simulink model "SimulationDemo"  (R2025b)
settings: Solver=ode4  StartTime=0.0  StopTime=200  FixedStep=0.02  RelTol=1e-3
InitFcn:
  | Initialization
model workspace (MAT data in the model file):
  actuatorInitial.Aileron_deg = 0
  actuatorInitial.Elevator_deg = 0
  actuatorInitial.Rudder_deg = 0
  contactParams.Kz_Npm = 5000
  contactParams.Cz_Nspm = 160
  contactParams.FrictionMu = 0.03
  contactParams.SlipSpeed_mps = 0.15
  contactParams.RampGain_1pm = 200
  contactParams.NormalScaleMax = 8
  contactParams.GroundPitch_rad = 0.0523598775598
  contactParams.PitchK_NmPerRad = -0.5
  contactParams.PitchC_NmPerRadps = -1
  contactParams.LateralFrictionMu = 1.5
  contactParams.RollK_NmPerRad = -8
  contactParams.RollC_NmPerRadps = -2.5
  contactParams.YawK_NmPerRad = -12
  contactParams.YawC_NmPerRadps = -4
  flightProtection.VMin_mps = 2
  flightProtection.VEps_mps = 0.001
  flightProtection.QGateBreakpoints_mps = [0 2 5]
  flightProtection.QGateTable = [0 0 1]
  flightProtection.BetaGateStartU_mps = 8
  flightProtection.BetaGateFullU_mps = 18
  initial.Heading = -2.35619449019
  initial.Roll = 0
  initial.Pitch = 0.0523598775598
  initial.Yaw = -2.35619449019
  initial.p = 0
  initial.q = 0.0001
  initial.r = 0.0001
  initial.u = 0.1
  initial.v = 0
  initial.w = 0.001
  initial.Altitude_MSL = 239
  initial.Altitude_AGL = 0
  initial.CGInertial.X = 0
  initial.CGInertial.Y = 0
  initial.CGInertial.Z = -239
  initial.Xe = [0 0 -239]
  initial.Mass.Empty = 1.67
  initial.Mass.Payload = 1.25
  initial.Mass.GrossTO = 2.92
  initial.Inertia = [0.026  0  0.0007; 0  0.072  0; 0.0007  0  0.096]
undefined symbols (not defined in the file): aeroData, aileronMax, aileronMin, dirPitch, dirRoll, dirThrottle, dirYaw, elevatorMax, elevatorMin, envActive, envCustomSource, envPresetSource, F, geometry, MIL, Moderate, pitchCh, pitchDB, propulsionData, rollCh, rollDB, throttleCh, throttleDB, uPitchMax, uPitchMin, uRollMax, uRollMin, uThrottleMax, uThrottleMin, uYawMax, uYawMin, yawCh, yawDB
libraries: simulink_extras x4, aerolibwind2 x3, aerolibasang x2, aerolibsim3d x2, aerolibadyn x1, matrix_library x1, sl3dlib x1, aerolibatmos2 x1, uavutilslib x1, sim3dlib x1
(part 1 of 2)
settings Model: DataDictionary=environmentData.sldd  Creator=klakhara  LastModifiedBy=klakhara
settings SolverCC: ODENIntegrationMethod=ode4

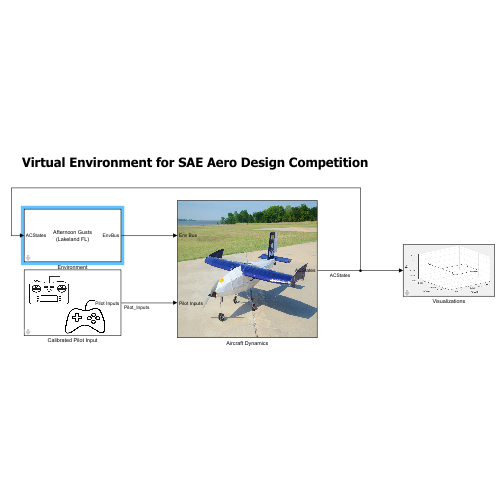
[thumbnail: Simulink's stored preview of the top-level diagram]
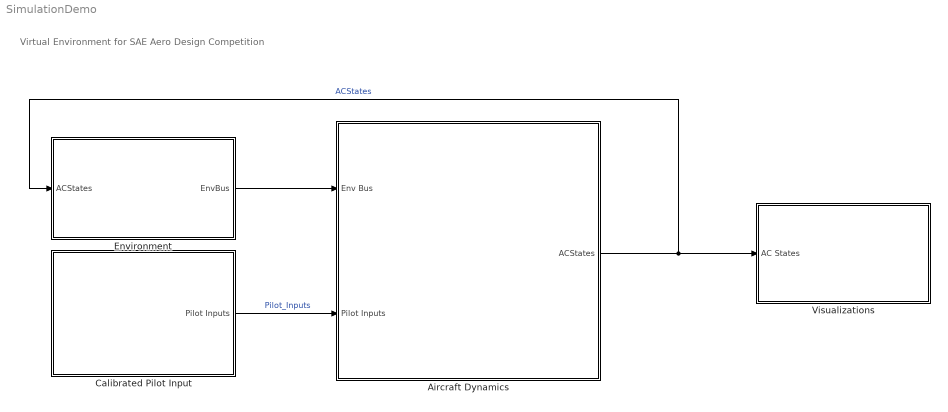
== system SimulationDemo ==
  note: Virtual Environment for SAE Aero Design Competition
  Aircraft Dynamics : Subsystem
      mask Display: image('Aircraft.jpg');
  Calibrated Pilot Input : Subsystem  mask{configName=0, joystickID=Joystick1}
      mask prompts: joystickID "Device ID:"
      mask TypeOptions joystickID: None | Joystick1 | Joystick2 | Joystick3 | Joystick4 | Joystick5 | Joystick6 | Joystick7 | Joystick8 | Joystick9 | Joystick10 | Joystick11 | Joystick12
      mask DialogControl DescGroupVar Prompt: Import calibration parameters to setup the calibreated input device
      mask DialogControl DescTextVar Prompt: Import your calibration configuration file:
      mask DialogControl loadConfig Prompt: Load file
      mask DialogControl ParameterGroupVar Prompt: Identify your Pilot Input Device:
      mask Display: image('Controller_Setup.jpg');
  Environment : Subsystem  mask(SAE Aero Environment){envPreset=Afternoon Gusts - Lakeland FL (2.0x), customName=VIT Vellore, customDescription=VIT Vellore, customMultiplier=1, customCompetitionSite=off, customLocationName=Custom Site, customCity=, customCountry=, customLatitude_deg=0, customLongitude_deg=0, customElevation_MSL_m=0, customAtmosphereElevation_MSL_m=0, customISADeviation_C=0, customTemperature_C=15, customPressure_Pa=101325, customDensity_kgm3=1.225, customWindShearSpeed_mps=0, customWindShearDirection_deg=0, customWindShearExponent=0.143, customTurbulenceOn=off, customTurbulenceSpeed_mps=0, customTurbulenceDirection_deg=0, customTurbulenceSigma_mps=0, customTurbulenceScale_m=205, customNoiseSeeds=[23341 23342 23343 23344], customGustEnableU=off, customGustEnableV=off, customGustEnableW=off, customGustAmplitude_mps=[0 0 0], customGustLength_m=[1 1 1], customGustStartTime_s=Inf, customGustStartAltitude_AGL_m=0}
      mask prompts: envPreset "Environment"; customName "Name"; customDescription "Description"; customMultiplier "Score multiplier"; customCompetitionSite "Competition site"; customLocationName "Location name"; customCity "City"; customCountry "Country or region"; customLatitude_deg "Latitude [deg]"; customLongitude_deg "Longitude [deg]"; customElevation_MSL_m "Elevation MSL [m]"; customAtmosphereElevation_MSL_m "Reference elevation [m]"; customISADeviation_C "ISA deviation [deg C]"; customTemperature_C "Temperature [deg C]"; customPressure_Pa "Pressure [Pa]"; customDensity_kgm3 "Density [kg/m^3]"; customWindShearSpeed_mps "Speed at 6 m [m/s]"; customWindShearDirection_deg "Direction [deg]"; customWindShearExponent "Power-law exponent"; customTurbulenceOn "Enable turbulence"; customTurbulenceSpeed_mps "Speed at 6 m [m/s]"; customTurbulenceDirection_deg "Direction [deg]"; customTurbulenceSigma_mps "Sigma [m/s]"; customTurbulenceScale_m "Scale length [m]"; customNoiseSeeds "Noise seeds [1x4]"; customGustEnableU "Enable U-axis gust"; customGustEnableV "Enable V-axis gust"; customGustEnableW "Enable W-axis gust"; customGustAmplitude_mps "Amplitude [u v w] m/s"; customGustLength_m "Length [dx dy dz] m"; customGustStartTime_s "Start time [s]"; customGustStartAltitude_AGL_m "Start altitude AGL [m]"
      mask help: Select a predefined environment or enter a complete custom environment definition.
      mask init:
      | EnvironmentMask.initialize(gcb);
      mask TypeOptions envPreset: Custom environment | Sea Level Standard (1.0x) | Aero Design West - Van Nuys CA (1.1x) | Aero Design East FL - Lakeland (1.2x) | Aero Design East TX - Fort Worth (1.3x) | Hot Day - Chennai India (1.5x) | Cold Windy Day - Toronto (1.6x) | Afternoon Gusts - Lakeland FL (2.0x) | High Altitude - Denver-type (2.5x)
      mask Callback envPreset: EnvironmentMask.selectionChanged(gcb);
      mask DialogControl Container1 Prompt: Environment source
      mask DialogControl Control1 Prompt: Predefined environments are loaded from environmentData.sldd.
      mask DialogControl envPreset Tooltip: Choose a catalog environment or enter a custom definition.
      mask DialogControl customGeneralTab Prompt: General
      mask DialogControl customName Tooltip: Name stored with simulation environment metadata.
      mask DialogControl customDescription Tooltip: Description stored with the environment.
      mask DialogControl customMultiplier Tooltip: Positive mission score multiplier.
      mask DialogControl customCompetitionSite Tooltip: Marks this environment as an official competition site.
      mask DialogControl customLocationTab Prompt: Location
      mask DialogControl customLocationName Tooltip: Airfield or test-site name.
      mask DialogControl customCity Tooltip: Location city.
      mask DialogControl customCountry Tooltip: Location country or region.
      mask DialogControl customLatitude_deg Tooltip: Geodetic latitude from -90 to 90 degrees.
      mask DialogControl customLongitude_deg Tooltip: Longitude from -180 to 180 degrees.
      mask DialogControl customElevation_MSL_m Tooltip: Site elevation above mean sea level.
      mask DialogControl customAtmosphereTab Prompt: Atmosphere
      mask DialogControl customAtmosphereElevation_MSL_m Tooltip: Elevation associated with the atmospheric measurements.
      mask DialogControl customISADeviation_C Tooltip: Temperature difference from ISA.
      mask DialogControl customTemperature_C Tooltip: Measured or specified air temperature.
      mask DialogControl customPressure_Pa Tooltip: Positive static air pressure.
      mask DialogControl customDensity_kgm3 Tooltip: Positive air density.
      mask DialogControl customWindTab Prompt: Wind shear
      mask DialogControl customWindShearSpeed_mps Tooltip: Nonnegative wind speed at the reference height.
      mask DialogControl customWindShearDirection_deg Tooltip: Meteorological direction clockwise from north.
      mask DialogControl customWindShearExponent Tooltip: Positive terrain-dependent shear exponent.
      mask DialogControl customTurbulenceTab Prompt: Turbulence
      mask DialogControl customTurbulenceOn Tooltip: Enable the Dryden turbulence model.
      mask DialogControl customTurbulenceSpeed_mps Tooltip: Nonnegative mean wind speed used by Dryden turbulence.
      mask DialogControl customTurbulenceDirection_deg Tooltip: Direction clockwise from north.
      mask DialogControl customTurbulenceSigma_mps Tooltip: RMS turbulence intensity.
      mask DialogControl customTurbulenceScale_m Tooltip: Positive medium/high-altitude scale length.
      mask DialogControl customNoiseSeeds Tooltip: Four nonnegative integer seeds.
      mask DialogControl customGustTab Prompt: Gust
      mask DialogControl customGustEnableU Tooltip: Enable longitudinal gust.
      mask DialogControl customGustEnableV Tooltip: Enable lateral gust.
      mask DialogControl customGustEnableW Tooltip: Enable vertical gust.
      mask DialogControl customGustAmplitude_mps Tooltip: Three gust velocity components.
      mask DialogControl customGustLength_m Tooltip: Three positive gust wavelengths.
      mask DialogControl customGustStartTime_s Tooltip: Nonnegative gust start time; use Inf to disable by time.
      mask DialogControl customGustStartAltitude_AGL_m Tooltip: Nonnegative gust onset altitude.
      mask Display:
      | try
      |     disp(EnvironmentMask.formatIconLabel(environmentName));
      | catch
      |     disp('Environment');
      | end
  Visualizations : Subsystem  mask{visualization=3D Animation, FlightParam=on}
      mask prompts: visualization "Trajectory visualization"; FlightParam "Plot flight parameters"
      mask Callback FlightParam:
      | scopeBlocks = find_system(gcb, 'LookUnderMasks', 'all', 'FollowLinks', 'off', 'MatchFilter', @Simulink.match.allVariants, 'BlockType', 'Scope');
      | scopeState = get_param(gcb, 'FlightParam');
      | for scopeIndex = 1:numel(scopeBlocks)
      |     set_param(scopeBlocks{scopeIndex}, 'OpenAtSimulationStart', scopeState, 'Open', scopeState);
      | end
      | clear scopeBlocks scopeState scopeIndex
      mask DialogControl DescTextVar Prompt: Select your visualization type and if you want to plot flight paramets in scope.
      mask Display:
      | % Get selected variant from mask
      | v = get_param(gcb, 'visualization');
      | 
      | 
      | % Choose image based on variant
      | switch v
      |     case '3D Animation'
      |         img = imread('3D_Animation.png');
      |         image(img);
      |         % axis off
      |         % axis image
      |     case "Unreal Engine"
      |         img = imread('Unreal_Engine.png');
      |         image(img);
      |         % axis off
      |         % axis image
      |     case 'Off'
      |         % No image
      | 
      | end
      | 
      | % Display image as block icon
  wires:
  Aircraft Dynamics/1(ACStates) -> Visualizations/1(AC States), Environment/1(ACStates)  "ACStates"
  Environment/1(EnvBus) -> Aircraft Dynamics/1(Env Bus)
  Calibrated Pilot Input/1(Pilot Inputs) -> Aircraft Dynamics/2(Pilot Inputs)  "Pilot_Inputs"

== system SimulationDemo/Aircraft Dynamics ==
  Env Bus : Inport
  Pilot Inputs : Inport  Port=2
  ACStates To Workspace : ToWorkspace  VariableName=ACStates  SaveFormat=Timeseries  SampleTime=-1
  Actuator Dynamics : Subsystem
  Bus Creator : BusCreator  Inputs=8
  Bus Selector : BusSelector  OutputSignals=Actuator deflections
  Equation of motion : EOM6DOFBodyQuat  xme_0=initial.Xe  Vm_0=[initial.u initial.v initial.w]  eul_0=[initial.Roll initial.Pitch initial.Yaw]  pm_0=[initial.p initial.q initial.r]  mass_0=initial.Mass.GrossTO  inertia=initial.Inertia
  Flight Parameters : Subsystem
  Forces & Moments : Subsystem
  Gain : Gain  Gain=[1, 1, -1]
  ACStates : Outport
  wires:
  Actuator Dynamics/1(Actuator_Deflections) -> Bus Creator/8, Forces & Moments/4(Pilot_Inputs)  "Actuator deflections"
  Bus Selector/1 -> Actuator Dynamics/1(Actuator_Command)  "<Actuator deflections>"
  Pilot Inputs/1 -> Bus Selector/1  "Pilot_Inputs"
  Forces & Moments/2(Moments) -> Equation of motion/2
  Forces & Moments/1(Forces) -> Equation of motion/1
  Flight Parameters/1(Flight_Parameters) -> Forces & Moments/2(Flight Params)
  Equation of motion/2 -> Gain/1
  Equation of motion/4 -> Bus Creator/4  "q"
  Gain/1 -> Bus Creator/2  "Xe"
  Env Bus/1 -> Flight Parameters/2(EnvirBus), Forces & Moments/3(Env Bus)
  Equation of motion/1 -> Bus Creator/1  "Ve"
  Equation of motion/5 -> Bus Creator/5  "DCM_be"
  Equation of motion/7 -> Bus Creator/7  "wb"
  Equation of motion/6 -> Bus Creator/6  "Vb"
  Equation of motion/3 -> Bus Creator/3  "Euler_angles"
  Bus Creator/1 -> Forces & Moments/1(States), Flight Parameters/1("AC States "), ACStates To Workspace/1, ACStates/1  "ACStates"

== system SimulationDemo/Calibrated Pilot Input ==
  Actuator scaling : Subsystem
  Bus Creator : BusCreator  Inputs=2
  PilotInput : BusCreator  Inputs=4
  Simulation 3D Joystick : sl3dlib/Simulation 3D/Hardware Interface/Simulation 3D Joystick  joyid=1  adjustports=on  forcefeed=off
  Terminator : Terminator
  Pilot Inputs : Outport
  wires:
  Bus Creator/1 -> Pilot Inputs/1
  Simulation 3D Joystick/1 -> Bus Creator/1, Actuator scaling/1(In1)  "Raw Inputs"
  Actuator scaling/2(Elevator) -> PilotInput/2  "Elevator"
  Simulation 3D Joystick/2 -> Terminator/1
  PilotInput/1 -> Bus Creator/2  "Actuator deflections"
  Actuator scaling/3(Rudder) -> PilotInput/3  "Rudder"
  Actuator scaling/4(Throttle) -> PilotInput/4  "Throttle"
  Actuator scaling/1(Aileron) -> PilotInput/1  "Aileron"

== system SimulationDemo/Environment ==
  ACStates : Inport
  AltitudeAGL : Sum  Inputs=+-
  AltitudeMSLValid : Saturate  UpperLimit=84852  LowerLimit=0
  AltitudePos : Gain  Gain=-1
  Bus Creator : BusCreator  Inputs=4
  Bus Creator1 : BusCreator  Inputs=2
  Bus Selector1 : BusSelector  OutputSignals=Xe,Ve,DCM_be
  Dot Product : DotProduct  OutDataTypeStr=Inherit: Inherit via internal rule
  Environment Source : Subsystem  Variant=on
  Mux : Mux  Inputs=3
  Reshape : Reshape  OutputDimensionality=Row vector (2-D)
  Selector2 : Selector  IndexMode=Zero-based  InputPortWidth=3  IndexOptions=Index vector (dialog)  Indices=2  OutputSizes=1
  Sqrt : Sqrt
  Temperature Adjusted Density : Subsystem
  "WGS84 Gravity Model  " : GravityWGS84  action=None
  Wind Models : Subsystem
  EnvBus : Outport  VectorParamsAs1DForOutWhenUnconnected=off
  wires:
  Wind Models/2(pg,qg,rg) -> Bus Creator1/2  "pqr_wind"
  Wind Models/1(ug,vg,wg) -> Bus Creator1/1  "uvw_wind"
  Bus Creator1/1 -> Bus Creator/4  "Vwind"
  Dot Product/1 -> Sqrt/1
  Sqrt/1 -> Wind Models/2(Airspeed)
  Bus Creator/1 -> EnvBus/1
  ACStates/1 -> Bus Selector1/1
  Bus Selector1/2 -> Dot Product/1, Dot Product/2  "<Ve>"
  Mux/1 -> Bus Creator/2, Reshape/1  "X"
  "WGS84 Gravity Model  "/1 -> Bus Creator/1  "g"
  Reshape/1 -> "WGS84 Gravity Model  "/1
  Bus Selector1/3 -> Wind Models/3(DCM)  "<DCM_be>"
  Bus Selector1/1 -> Selector2/1  "<Xe>"
  Selector2/1 -> AltitudePos/1
  AltitudeAGL/1 -> Wind Models/1(Altitude)
  AltitudePos/1 -> AltitudeMSLValid/1
  AltitudeMSLValid/1 -> Mux/3, AltitudeAGL/1, Temperature Adjusted Density/2(Height)
  Temperature Adjusted Density/1(rho) -> Bus Creator/3
  Environment Source/1(Latitude_deg) -> Mux/1  "Latitude_deg"
  Environment Source/2(Longitude_deg) -> Mux/2  "Longitude_deg"
  Environment Source/4(Elevation_MSL_m) -> AltitudeAGL/2  "Elevation_MSL_m"
  Environment Source/3(ISA_Deviation_C) -> Temperature Adjusted Density/1(ISA_Deviation_C)  "ISA_Deviation_C"

== system SimulationDemo/Visualizations ==
  AC States : Inport
  "Flight parameters " : Subsystem  Variant=on  EmptyChoice=on
  Trajectory Visualization : Subsystem  Variant=on  EmptyChoice=on
  wires:
  AC States/1 -> Trajectory Visualization/1(AC States), "Flight parameters "/1(In1)

== system SimulationDemo/Aircraft Dynamics/Actuator Dynamics ==
  Actuator_Command : Inport
  Aileron_Command_Limit : Saturate  UpperLimit=geometry.AileronLimit(2)  LowerLimit=geometry.AileronLimit(1)
  Aileron_Deflection_Limit : Saturate  UpperLimit=geometry.AileronLimit(2)  LowerLimit=geometry.AileronLimit(1)
  Aileron_Lag_0p05s : StateSpace  A=-20  B=20  D=0  InitialCondition=actuatorInitial.Aileron_deg
  Aileron_Rate_300dps : RateLimiter  RisingSlewLimit=300  FallingSlewLimit=-300  InitialCondition=actuatorInitial.Aileron_deg
  Command_Select : BusSelector  OutputSignals=Aileron,Elevator,Rudder,Throttle
  Deflection_Bus : BusCreator  Inputs=4
  Elevator_Command_Limit : Saturate  UpperLimit=geometry.ElevatorLimit(2)  LowerLimit=geometry.ElevatorLimit(1)
  Elevator_Deflection_Limit : Saturate  UpperLimit=geometry.ElevatorLimit(2)  LowerLimit=geometry.ElevatorLimit(1)
  Elevator_Lag_0p05s : StateSpace  A=-20  B=20  D=0  InitialCondition=actuatorInitial.Elevator_deg
  Elevator_Rate_300dps : RateLimiter  RisingSlewLimit=300  FallingSlewLimit=-300  InitialCondition=actuatorInitial.Elevator_deg
  Rudder_Command_Limit : Saturate  UpperLimit=geometry.RudderLimit(2)  LowerLimit=geometry.RudderLimit(1)
  Rudder_Deflection_Limit : Saturate  UpperLimit=geometry.RudderLimit(2)  LowerLimit=geometry.RudderLimit(1)
  Rudder_Lag_0p05s : StateSpace  A=-20  B=20  D=0  InitialCondition=actuatorInitial.Rudder_deg
  Rudder_Rate_300dps : RateLimiter  RisingSlewLimit=300  FallingSlewLimit=-300  InitialCondition=actuatorInitial.Rudder_deg
  Actuator_Deflections : Outport
  wires:
  Actuator_Command/1 -> Command_Select/1
  Aileron_Command_Limit/1 -> Aileron_Lag_0p05s/1
  Command_Select/1 -> Aileron_Command_Limit/1  "<Aileron>"
  Command_Select/2 -> Elevator_Command_Limit/1  "<Elevator>"
  Command_Select/3 -> Rudder_Command_Limit/1  "<Rudder>"
  Elevator_Command_Limit/1 -> Elevator_Lag_0p05s/1
  Command_Select/4 -> Deflection_Bus/4  "<Throttle>"
  Rudder_Command_Limit/1 -> Rudder_Lag_0p05s/1
  Aileron_Lag_0p05s/1 -> Aileron_Rate_300dps/1
  Elevator_Lag_0p05s/1 -> Elevator_Rate_300dps/1
  Rudder_Lag_0p05s/1 -> Rudder_Rate_300dps/1
  Aileron_Rate_300dps/1 -> Aileron_Deflection_Limit/1
  Elevator_Rate_300dps/1 -> Elevator_Deflection_Limit/1
  Rudder_Rate_300dps/1 -> Rudder_Deflection_Limit/1
  Elevator_Deflection_Limit/1 -> Deflection_Bus/2  "Elevator"
  Aileron_Deflection_Limit/1 -> Deflection_Bus/1  "Aileron"
  Rudder_Deflection_Limit/1 -> Deflection_Bus/3  "Rudder"
  Deflection_Bus/1 -> Actuator_Deflections/1

== system SimulationDemo/Aircraft Dynamics/Flight Parameters ==
  "AC States " : Inport
  EnvirBus : Inport  Port=2
  Bus Creator : BusCreator  Inputs=6
  Bus Selector1 : BusSelector  OutputSignals=rho
  Bus Selector2 : BusSelector  OutputSignals=Vb
  Bus Selector3 : BusSelector  OutputSignals=wb
  Bus Selector4 : BusSelector  OutputSignals=Vwind.uvw_wind,Vwind.pqr_wind
  Flight Parameters To Workspace : ToWorkspace  VariableName=FlightParameters  SaveFormat=Timeseries  SampleTime=-1
  "Incidence, Sideslip, & Airspeed" : aerolibasang/Incidence, Sideslip, & Airspeed
  Radians to Degrees : simulink_extras/Transformations/Radians to Degrees
  Radians to Degrees1 : simulink_extras/Transformations/Radians to Degrees
  Subsystem : Subsystem
      settings: PortSchema="{\"entries\":[{\"content\":{\"sides\":[{\"content\":{\"connectorIds\":[\"In1\",\"In2\"]},\"type\":\"ConnectorPlacement.EquallySpacedRectSide\",\"uuid\":\"5a143d0f-2436-4fb0-bb97-2c4984d07975\"},{\"content\":{\"connectorIds\":[\"Out1\"],\"side\":\"RIGHT\"},\"type\":\"ConnectorPlacement.EquallySpacedRectSide\",\"uuid\":\"8d58a2ee-82c7-4615-9bab-8cc4c0d46ad5\"},{\"content\":{\"connectorIds\":[\"In3\"],\"side\":\"TOP\"},\"type\":\"ConnectorPlacement.EquallySpacedRectSide\",\"uuid\":\"18f756c1-07a2-4df5-83f0-d5c22876817a\"}]},\"type\":\"ConnectorPlacement.EquallySpacedConnector\",\"uuid\":\"42d60932-45cf-443a-a7ca-3ff9305e2569\"}],\"packageUris\":[\"http://schema.mathworks.com/mf0/Connector/R2020b\"],\"version\":\"1.0\"}"
  Sum2 : Sum  InputSameDT=on  SaturateOnIntegerOverflow=on  OutDataTypeStr=Inherit: Same as first input
  Sum4 : Sum  Inputs=+-|  InputSameDT=on  SaturateOnIntegerOverflow=on  OutDataTypeStr=Inherit: Same as first input
  Vrel_safe : Subsystem
  Flight_Parameters : Outport  VectorParamsAs1DForOutWhenUnconnected=off
  wires:
  "AC States "/1 -> Bus Selector2/1, Bus Selector3/1
  Sum2/1 -> Bus Creator/5  "pqr_tot"
  Sum4/1 -> Vrel_safe/1(Vrel)  "Vrel"
  Bus Selector3/1 -> Sum2/2  "<wb>"
  EnvirBus/1 -> Bus Selector1/1, Bus Selector4/1
  Bus Selector2/1 -> Sum4/1  "<Vb>"
  Bus Selector4/2 -> Sum2/1  "<pqr_wind>"
  Bus Selector4/1 -> Sum4/2  "<uvw_wind>"
  "Incidence, Sideslip, & Airspeed"/3 -> Subsystem/3(TAS), Bus Creator/4  "TAS"
  "Incidence, Sideslip, & Airspeed"/1 -> Radians to Degrees/1
  "Incidence, Sideslip, & Airspeed"/2 -> Radians to Degrees1/1
  Vrel_safe/1(Vrel_safe) -> Subsystem/1(Vrel_safe), "Incidence, Sideslip, & Airspeed"/1, Bus Creator/1  "Vrel"
  Bus Selector1/1 -> Subsystem/2(<rho>)  "<rho>"
  Subsystem/1(q) -> Bus Creator/6  "dynamic Pressure"
  Radians to Degrees/1 -> Bus Creator/2  "alpha"
  Radians to Degrees1/1 -> Bus Creator/3  "beta"
  Bus Creator/1 -> Flight Parameters To Workspace/1, Flight_Parameters/1

== system SimulationDemo/Aircraft Dynamics/Forces & Moments ==
  note: Forces & Moments
      | 1. Gravitational Forces
      | 2. Aerodynamic Forces & Moments
      | 3. Propulsion Forces & Moments
  States : Inport
  Flight Params : Inport  Port=2
  Env Bus : Inport  Port=3
  Pilot_Inputs : Inport  Port=4
  Aerodynamic Forces & Moments : Subsystem
  Bus Selector : BusSelector  OutputSignals=g
  Bus Selector1 : BusSelector  OutputSignals=Xe,DCM_be,Vb
  Contact Forces & Moments : Subsystem
  Gravitational Forces : Subsystem
  Propulsion Forces & Moments : Subsystem
  Sum : Sum  Inputs=++++
  Sum1 : Sum  Inputs=+++
  Forces : Outport
  Moments : Outport  Port=2
  wires:
  Bus Selector1/3 -> Contact Forces & Moments/4(Vb)  "<Vb>"
  Contact Forces & Moments/1(F_Contact) -> Sum/4
  Bus Selector1/1 -> Contact Forces & Moments/2(Xe)  "<Xe>"
  Bus Selector1/2 -> Gravitational Forces/1(DCM)  "<DCM_be>"
  Sum1/1 -> Moments/1  "Moments"
  Sum/1 -> Forces/1  "Forces"
  Propulsion Forces & Moments/1(Forces_Propulsion) -> Sum/3  "F_Prop"
  Aerodynamic Forces & Moments/1(Forces_aero) -> Sum/2  "F_Aero"
  Gravitational Forces/1(Fgrav) -> Sum/1, Contact Forces & Moments/3(F_Gravity)  "F_Gravity"
  Bus Selector/1 -> Gravitational Forces/2(g)  "<g>"
  States/1 -> Bus Selector1/1, Contact Forces & Moments/1(States)  "States"
  Env Bus/1 -> Propulsion Forces & Moments/2(EnvBus), Bus Selector/1
  Flight Params/1 -> Aerodynamic Forces & Moments/1(Flight Params)
  Propulsion Forces & Moments/2(Moments_Propulsion) -> Sum1/2  "M_Prop"
  Pilot_Inputs/1 -> Aerodynamic Forces & Moments/2(Pilot_Input), Propulsion Forces & Moments/1(Pilot Inputs)
  Aerodynamic Forces & Moments/2(Moments_aero) -> Sum1/1  "M_Aero"
  Contact Forces & Moments/2(M_Contact) -> Sum1/3  "M_Contact"

== system SimulationDemo/Calibrated Pilot Input/Actuator scaling ==
  In1 : Inport
  Aileron Scaling : Subsystem
  Demux : Demux
  Elevator Scaling : Subsystem
  Rudder Scaling : Subsystem
  Selector : Selector  InputPortWidth=8  IndexOptions=Index vector (dialog)  Indices=[rollCh pitchCh yawCh throttleCh]  OutputSizes=1
  Throttle Scaling : Subsystem
  Aileron : Outport
  Elevator : Outport  Port=2
  Rudder : Outport  Port=3
  Throttle : Outport  Port=4
  wires:
  In1/1 -> Selector/1
  Rudder Scaling/1(actuator deflection) -> Rudder/1
  Demux/3 -> Rudder Scaling/1(raw signal)  "Yaw"
  Demux/1 -> Aileron Scaling/1(raw signal)  "roll"
  Selector/1 -> Demux/1
  Elevator Scaling/1(actuator deflection) -> Elevator/1
  Demux/4 -> Throttle Scaling/1(raw signal)  "Throttle"
  Demux/2 -> Elevator Scaling/1(raw signal)  "Pitch"
  Aileron Scaling/1(actuator deflection) -> Aileron/1
  Throttle Scaling/1(actuator deflection) -> Throttle/1

== system SimulationDemo/Environment/Environment Source ==
  note: 1) Add Subsystem or Model blocks as valid variant choices.
      | 2) You cannot connect blocks at this level. At simulation, connectivity is automatically
      | determined, based on the active variant and port name matching.
  Custom Environment Parameters : Subsystem  VariantControl=environmentSourceMode == 1
  Preset Environment Parameters : Subsystem  VariantControl=environmentSourceMode == 2
  Latitude_deg : Outport
  Longitude_deg : Outport  Port=2
  ISA_Deviation_C : Outport  Port=3
  Elevation_MSL_m : Outport  Port=4

== system SimulationDemo/Environment/Temperature Adjusted Density ==
  ISA_Deviation_C : Inport
  Height : Inport  Port=2
  Adjusted Temperature : Sum
  COESA Atmosphere Model : aerolibatmos2/COESA Atmosphere Model  units=Metric (MKS)  spec=1976 COESA-extended U.S. Standard Atmosphere  model=Profile  profile_var=High temperature  profile_percent=1%  profile_alt=5 km (16404 ft)  envelope_var=High temperature  envelope_percent=1%  action=Warning
  Density Correction : Product  Inputs=**/
  Temperature Guard : Saturate  UpperLimit=inf  LowerLimit=1
  Terminator2 : Terminator
  Terminator3 : Terminator
  rho : Outport
  wires:
  Adjusted Temperature/1 -> Temperature Guard/1
  COESA Atmosphere Model/3 -> Terminator2/1  "ps"
  COESA Atmosphere Model/1 -> Density Correction/2, Adjusted Temperature/2  "T"
  COESA Atmosphere Model/4 -> Density Correction/1  "rho"
  COESA Atmosphere Model/2 -> Terminator3/1  "a"
  Temperature Guard/1 -> Density Correction/3
  Height/1 -> COESA Atmosphere Model/1
  Density Correction/1 -> rho/1  "rho"
  ISA_Deviation_C/1 -> Adjusted Temperature/1

== system SimulationDemo/Environment/Wind Models ==
  Altitude : Inport  Unit=meter
  Airspeed : Inport  Port=2  Unit=m/s
  DCM : Inport  Port=3
  "DCM " : InportShadow  Port=3
  Discrete Wind Gust Model : aerolibwind2/Discrete Wind Gust Model  units=Metric (MKS)  Gx=off  Gy=on  Gz=off  t_0=envActive.Gust.StartTime_s  d_m=envActive.Gust.Length_m  v_m=envActive.Gust.Amplitude_mps
  Dryden Wind Turbulence Model (Continuous (+q -r)) : aerolibwind2/Dryden Wind Turbulence Model  (Continuous (+q -r))  units=Metric (MKS)  spec=MIL-F-8785C  model=Continuous Dryden (+q -r)  W20=envActive.Turbulence.Speed_6m_mps  Wdeg=envActive.Turbulence.Direction_deg  TurbProb=10^-3 - Moderate  L_high=envActive.Turbulence.Scale_Lu_m  Wingspan=geometry.Span  ts=0.5  Seed=envActive.Turbulence.NoiseSeeds  T_on=on
  Sum : Sum  Inputs=+++  InputSameDT=on  SaturateOnIntegerOverflow=on  OutDataTypeStr=Inherit: Same as first input
  Wind Shear Model : aerolibwind2/Wind Shear Model  units=Metric (MKS)  phase=Category C - Terminal Flight Phase  W_20=envActive.WindShear.Speed_6m_mps  Wdeg=envActive.WindShear.Direction_deg
  ug,vg,wg : Outport  Unit=m/s  VectorParamsAs1DForOutWhenUnconnected=off
  pg,qg,rg : Outport  Port=2  Unit=rad/second  VectorParamsAs1DForOutWhenUnconnected=off
  wires:
  "DCM "/1 -> Dryden Wind Turbulence Model (Continuous (+q -r))/3
  Wind Shear Model/1 -> Sum/1
  Dryden Wind Turbulence Model (Continuous (+q -r))/1 -> Sum/2
  Discrete Wind Gust Model/1 -> Sum/3
  Sum/1 -> ug,vg,wg/1
  DCM/1 -> Wind Shear Model/2
  Airspeed/1 -> Dryden Wind Turbulence Model (Continuous (+q -r))/2, Discrete Wind Gust Model/1
  Dryden Wind Turbulence Model (Continuous (+q -r))/2 -> pg,qg,rg/1
  Altitude/1 -> Dryden Wind Turbulence Model (Continuous (+q -r))/1, Wind Shear Model/1

== system SimulationDemo/Visualizations/Flight parameters  ==
  In1 : Inport
  Scope Plot : Subsystem  TreatAsAtomicUnit=on  VariantControl=FlightParam ==1

== system SimulationDemo/Visualizations/Trajectory Visualization ==
  AC States : Inport
  3D Animation : Subsystem  VariantControl="visualization == \"3D Animation\""
      mask Display: image('3D_Animation.png');
  Unreal Engine : Subsystem  VariantControl="visualization == \"Unreal Engine\""
      mask Display: image('Unreal_Engine.png');

== system SimulationDemo/Aircraft Dynamics/Flight Parameters/Subsystem ==
  note: Note: 1D lookup table here is used as a switch to protect dynamic pressure for speed below 2 m/sec and gradually ramps up till 5 m/sec.
  Vrel_safe : Inport
  <rho> : Inport  Port=2
  TAS : Inport  Port=3
  1-D Lookup Table : Lookup_n-D  NumberOfTableDimensions=1  BreakpointsForDimension1=flightProtection.QGateBreakpoints_mps  Table=flightProtection.QGateTable  InterpMethod=Flat  ExtrapMethod=Clip  InternalRulePriority=Speed  RndMeth=Simplest
  Dynamic Pressure : aerolibasang/Dynamic Pressure
  Product : Product
  q : Outport
  wires:
  Vrel_safe/1 -> Dynamic Pressure/1
  <rho>/1 -> Dynamic Pressure/2
  1-D Lookup Table/1 -> Product/1
  Dynamic Pressure/1 -> Product/2
  Product/1 -> q/1
  TAS/1 -> 1-D Lookup Table/1

== system SimulationDemo/Aircraft Dynamics/Flight Parameters/Vrel_safe ==
  Vrel : Inport
  Mux_Vrel_safe : Mux  Inputs=3
  Split_Vrel : Demux  Outputs=3
  V_denom : MinMax  Function=max  Inputs=2
  V_min : Constant  Value=flightProtection.VMin_mps
  V_safe : MinMax  Function=max  Inputs=2
  eps_V : Constant  Value=flightProtection.VEps_mps
  scale : Product  Inputs=*/
  speed_sq : Sum  Inputs=+++
  sqrt_speed : Math  Operator=sqrt  SignedPower=on  RndMeth=Zero
  u_safe : Product
  u_sq : Product
  v_safe : Product
  v_sq : Product
  w_safe : Product
  w_sq : Product
  Vrel_safe : Outport
  wires:
  speed_sq/1 -> sqrt_speed/1  "V_mag_sq"
  Vrel/1 -> Split_Vrel/1
  u_sq/1 -> speed_sq/1
  w_sq/1 -> speed_sq/3
  Split_Vrel/1 -> u_sq/2, u_sq/1, u_safe/1  "u_rel"
  Split_Vrel/2 -> v_sq/1, v_sq/2, v_safe/1  "v_rel"
  v_sq/1 -> speed_sq/2
  Split_Vrel/3 -> w_safe/1, w_sq/2, w_sq/1  "w_rel"
  V_min/1 -> V_safe/2
  sqrt_speed/1 -> V_safe/1, V_denom/1  "V_mag"
  eps_V/1 -> V_denom/2
  V_safe/1 -> scale/1  "V_safe_mag"
  V_denom/1 -> scale/2
  u_safe/1 -> Mux_Vrel_safe/1  "u_rel_safe"
  scale/1 -> v_safe/2, w_safe/2, u_safe/2  "V_guard_scale"
  w_safe/1 -> Mux_Vrel_safe/3  "w_rel_safe"
  v_safe/1 -> Mux_Vrel_safe/2  "v_rel_safe"
  Mux_Vrel_safe/1 -> Vrel_safe/1  "Vrel_safe"

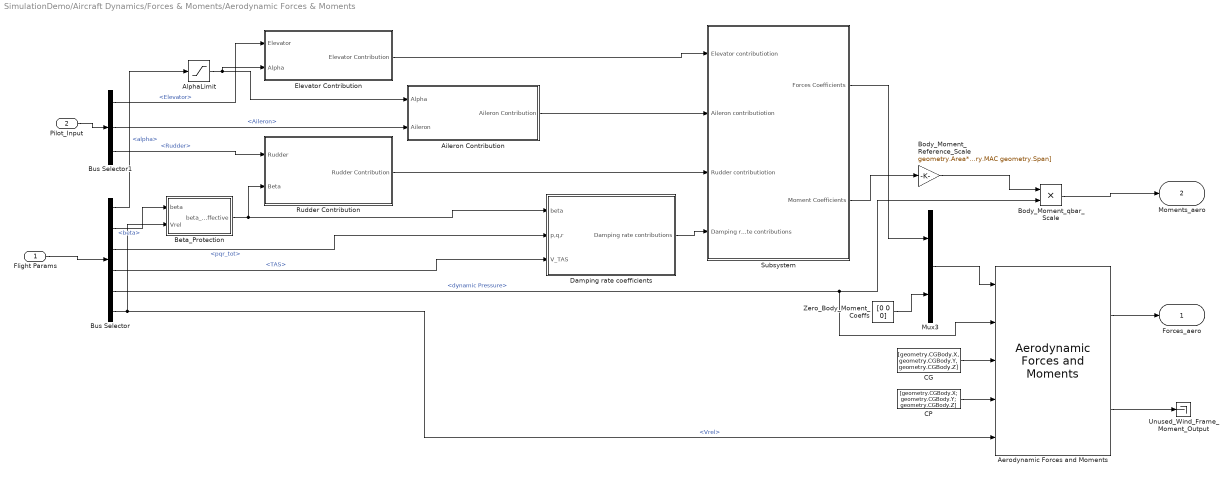
== system SimulationDemo/Aircraft Dynamics/Forces & Moments/Aerodynamic Forces & Moments ==
  Flight Params : Inport
  Pilot_Input : Inport  Port=2
  "Aerodynamic Forces and Moments " : aerolibadyn/Aerodynamic Forces and Moments   inputAxes=Wind  outputForceAxes=Body  outputMomentAxes=Body  S=geometry.Area  b=geometry.Span  cbar=geometry.MAC
  Aileron Contribution : Subsystem
  AlphaLimit : Saturate  UpperLimit=aeroData.validAlphaRange_deg(2)  LowerLimit=aeroData.validAlphaRange_deg(1)
  Beta_Protection : Subsystem
  Body_Moment_Reference_Scale : Gain  Gain=geometry.Area*[geometry.Span geometry.MAC geometry.Span]
  Body_Moment_qbar_Scale : Product
  Bus Selector : BusSelector  OutputSignals=alpha,beta,pqr_tot,TAS,dynamic Pressure,Vrel
  Bus Selector1 : BusSelector  OutputSignals=Elevator,Aileron,Rudder
  CG : Constant  Value="[geometry.CGBody.X, geometry.CGBody.Y,  geometry.CGBody.Z]"
  CP : Constant  Value=[geometry.CGBody.X; geometry.CGBody.Y; geometry.CGBody.Z]
  Damping rate coefficients : Subsystem
  Elevator Contribution : Subsystem
  Mux3 : Mux  Inputs=2
  Rudder Contribution : Subsystem
  Subsystem : Subsystem
  Unused_Wind_Frame_Moment_Output : Terminator
  Zero_Body_Moment_Coeffs : Constant  Value=[0 0 0]
  Forces_aero : Outport
  Moments_aero : Outport  Port=2
  wires:
  "Aerodynamic Forces and Moments "/2 -> Unused_Wind_Frame_Moment_Output/1
  Bus Selector/1 -> AlphaLimit/1  "<alpha>"
  Flight Params/1 -> Bus Selector/1
  Bus Selector/4 -> Damping rate coefficients/3(V_TAS)  "<TAS>"
  AlphaLimit/1 -> Elevator Contribution/2(Alpha), Aileron Contribution/1(Alpha)
  Bus Selector/2 -> Beta_Protection/1(beta)  "<beta>"
  Bus Selector/3 -> Damping rate coefficients/2(p,q,r)  "<pqr_tot>"
  Elevator Contribution/1(Elevator Contribution) -> Subsystem/1(Elevator contributiotion)
  Bus Selector/5 -> Body_Moment_qbar_Scale/2, "Aerodynamic Forces and Moments "/2  "<dynamic Pressure>"
  Bus Selector/6 -> Beta_Protection/2(Vrel), "Aerodynamic Forces and Moments "/5  "<Vrel>"
  CG/1 -> "Aerodynamic Forces and Moments "/3
  CP/1 -> "Aerodynamic Forces and Moments "/4
  Pilot_Input/1 -> Bus Selector1/1
  Bus Selector1/1 -> Elevator Contribution/1(Elevator)  "<Elevator>"
  Bus Selector1/2 -> Aileron Contribution/2(Aileron)  "<Aileron>"
  Bus Selector1/3 -> Rudder Contribution/1(Rudder)  "<Rudder>"
  Aileron Contribution/1(Aileron Contribution) -> Subsystem/2(Aileron contributiotion)
  Rudder Contribution/1("Rudder Contribution ") -> Subsystem/3(Rudder contributiotion)
  Damping rate coefficients/1(Damping rate contributions) -> Subsystem/4(Damping rate contributions)
  Subsystem/1(Forces Coefficients) -> Mux3/1
  Mux3/1 -> "Aerodynamic Forces and Moments "/1
  "Aerodynamic Forces and Moments "/1 -> Forces_aero/1
  Beta_Protection/1(beta_effective) -> Damping rate coefficients/1(beta), Rudder Contribution/2(Beta)
  Zero_Body_Moment_Coeffs/1 -> Mux3/2
  Subsystem/2(Moment Coefficients) -> Body_Moment_Reference_Scale/1
  Body_Moment_Reference_Scale/1 -> Body_Moment_qbar_Scale/1
  Body_Moment_qbar_Scale/1 -> Moments_aero/1

== system SimulationDemo/Aircraft Dynamics/Forces & Moments/Contact Forces & Moments ==
  States : Inport
  Xe : Inport  Port=2
  F_Gravity : Inport  Port=3
  Vb : Inport  Port=4
  Contact_Force_Total : Sum
  Ground_Contact_Switch : Switch  Criteria=u2 > Threshold  Threshold=initial.Mass.GrossTO*9.80665/contactParams.Kz_Npm
  Normal_Friction_Forces : Subsystem
  Pitch_Contact_Moment : Subsystem
  Select_Ze : Selector  InputPortWidth=3  IndexOptions=Index vector (dialog)  Indices=[3]  OutputSizes=1
  Zero_Force : Constant  Value=[0;0;0]
  F_Contact : Outport
  M_Contact : Outport  Port=2
  wires:
  Pitch_Contact_Moment/1(M_Contact) -> M_Contact/1  "M_Contact"
  States/1 -> Normal_Friction_Forces/4(States), Pitch_Contact_Moment/1(States)
  Normal_Friction_Forces/2(F_Contact_Friction) -> Contact_Force_Total/2
  Normal_Friction_Forces/1(F_Contact_Normal) -> Contact_Force_Total/1
  Vb/1 -> Normal_Friction_Forces/3(Vb)
  F_Gravity/1 -> Normal_Friction_Forces/2(F_Gravity)
  Contact_Force_Total/1 -> Ground_Contact_Switch/3
  Ground_Contact_Switch/1 -> F_Contact/1
  Zero_Force/1 -> Ground_Contact_Switch/1
  Select_Ze/1 -> Normal_Friction_Forces/1(Ze), Ground_Contact_Switch/2
  Xe/1 -> Select_Ze/1

== system SimulationDemo/Aircraft Dynamics/Forces & Moments/Gravitational Forces ==
  DCM : Inport
  g : Inport  Port=2  Unit=m/s^2
  Gross TO mass : Gain  Gain=initial.Mass.GrossTO  SaturateOnIntegerOverflow=on  OutDataTypeStr=Inherit: Same as input  ParamDataTypeStr=Inherit: Same as input
  Inertial to Body : Product  Multiplication=Matrix(*)  InputSameDT=on  SaturateOnIntegerOverflow=on  OutDataTypeStr=Inherit: Same as first input
  Reshape : Reshape  OutputDimensionality=Column vector (2-D)
  Reshape1 : Reshape
  Fgrav : Outport  Unit=N  VectorParamsAs1DForOutWhenUnconnected=off
  wires:
  Inertial to Body/1 -> Reshape1/1
  g/1 -> Gross TO mass/1
  DCM/1 -> Inertial to Body/1
  Gross TO mass/1 -> Reshape/1
  Reshape/1 -> Inertial to Body/2
  Reshape1/1 -> Fgrav/1

== system SimulationDemo/Aircraft Dynamics/Forces & Moments/Propulsion Forces & Moments ==
  Pilot Inputs : Inport
  EnvBus : Inport  Port=2
  Density Correction : Subsystem
  Gain : Gain
  Product : Product
  Subsystem : Subsystem
      settings: PortSchema="{\"entries\":[{\"content\":{\"sides\":[{\"content\":{\"connectorIds\":[\"Out1\"]},\"type\":\"ConnectorPlacement.EquallySpacedRectSide\",\"uuid\":\"fb30b856-b505-4c52-9be5-f51b9b4f9b3d\"},{\"content\":{\"side\":\"RIGHT\"},\"type\":\"ConnectorPlacement.EquallySpacedRectSide\",\"uuid\":\"6b49ea0c-e042-48c7-9a23-d0c81f552445\"},{\"content\":{\"connectorIds\":[\"In1\"],\"side\":\"TOP\"},\"type\":\"ConnectorPlacement.EquallySpacedRectSide\",\"uuid\":\"9dc7e958-cdfa-43a2-9a4f-607dc953e274\"}]},\"type\":\"ConnectorPlacement.EquallySpacedConnector\",\"uuid\":\"2adf19d2-e141-4d29-811e-0d4bf7e85bad\"}],\"packageUris\":[\"http://schema.mathworks.com/mf0/Connector/R2020b\"],\"version\":\"1.0\"}"
  Subsystem1 : Subsystem
  Subsystem2 : Subsystem
  Forces_Propulsion : Outport
  Moments_Propulsion : Outport  Port=2
  wires:
  Gain/1 -> Forces_Propulsion/1, Subsystem/1(Forces)
  Product/1 -> Subsystem1/1(Density corrected Thrust)
  Subsystem1/1(Forces_Propulsion) -> Gain/1
  Subsystem/1(Moments) -> Moments_Propulsion/1  "Moments_Propulsion"
  EnvBus/1 -> Density Correction/1(In1)
  Density Correction/1(Out1) -> Product/2
  Pilot Inputs/1 -> Subsystem2/1(Pilot_Inputs)  "Pilot_Inputs"
  Subsystem2/1(Motor_Prop_Thrust) -> Product/1

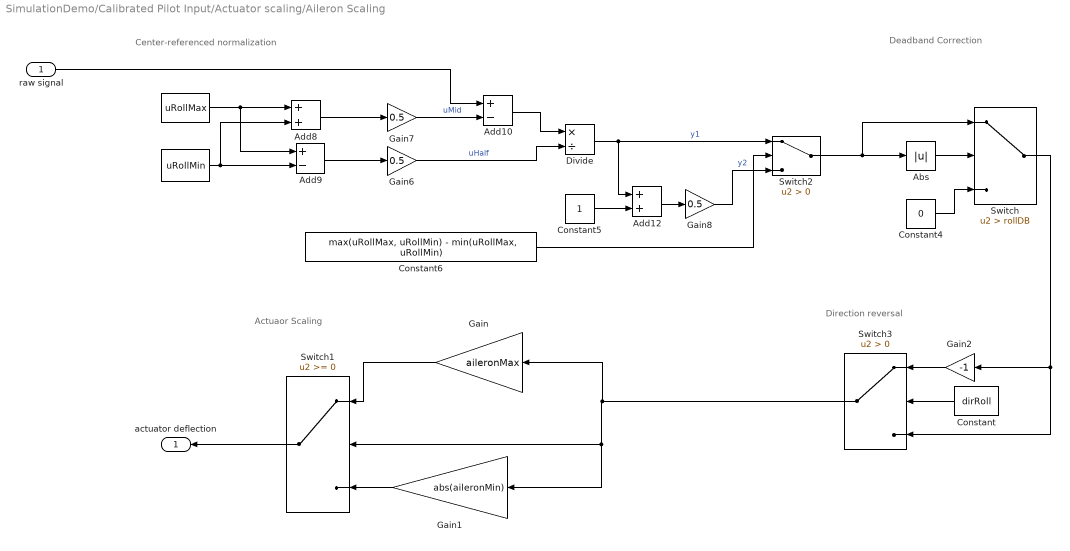
== system SimulationDemo/Calibrated Pilot Input/Actuator scaling/Aileron Scaling ==
  note: Direction reversal
  note: Center-referenced normalization
  note: Deadband Correction
  note: Actuaor Scaling
  raw signal : Inport
  " " : Constant  Value=uRollMin
  "   " : Constant  Value=uRollMax
  Abs : Abs  SaturateOnIntegerOverflow=off
  Add10 : Sum  Inputs=+-
  Add12 : Sum
  Add8 : Sum
  Add9 : Sum  Inputs=+-
  Constant : Constant  Value=dirRoll
  Constant4 : Constant  Value=0
  Constant5 : Constant
  Constant6 : Constant  Value=max(uRollMax, uRollMin) - min(uRollMax, uRollMin)
  Divide : Product  Inputs=*/
  Gain : Gain  Gain=aileronMax
  Gain1 : Gain  Gain=abs(aileronMin)
  Gain2 : Gain  Gain=-1
  Gain6 : Gain  Gain=0.5
  Gain7 : Gain  Gain=0.5
  Gain8 : Gain  Gain=0.5
  Switch : Switch  Criteria=u2 > Threshold  Threshold=rollDB  SaturateOnIntegerOverflow=off  InputSameDT=off
  Switch1 : Switch  SaturateOnIntegerOverflow=off  InputSameDT=off
  Switch2 : Switch  Criteria=u2 > Threshold  SaturateOnIntegerOverflow=off  InputSameDT=off
  Switch3 : Switch  Criteria=u2 > Threshold  SaturateOnIntegerOverflow=off  InputSameDT=off
  actuator deflection : Outport
  wires:
  Add9/1 -> Gain6/1
  "   "/1 -> Add9/1, Add8/1
  Add8/1 -> Gain7/1
  " "/1 -> Add8/2, Add9/2
  raw signal/1 -> Add10/1
  Gain7/1 -> Add10/2  "uMid"
  Add10/1 -> Divide/1
  Gain6/1 -> Divide/2  "uHalf"
  Switch1/1 -> actuator deflection/1
  Divide/1 -> Add12/1, Switch2/1  "y1"
  Constant5/1 -> Add12/2
  Add12/1 -> Gain8/1
  Constant6/1 -> Switch2/2
  Gain8/1 -> Switch2/3  "y2"
  Abs/1 -> Switch/2
  Constant4/1 -> Switch/3
  Switch/1 -> Gain2/1, Switch3/3
  Gain/1 -> Switch1/1
  Gain1/1 -> Switch1/3
  Gain2/1 -> Switch3/1
  Switch3/1 -> Gain1/1, Switch1/2, Gain/1
  Constant/1 -> Switch3/2
  Switch2/1 -> Switch/1, Abs/1

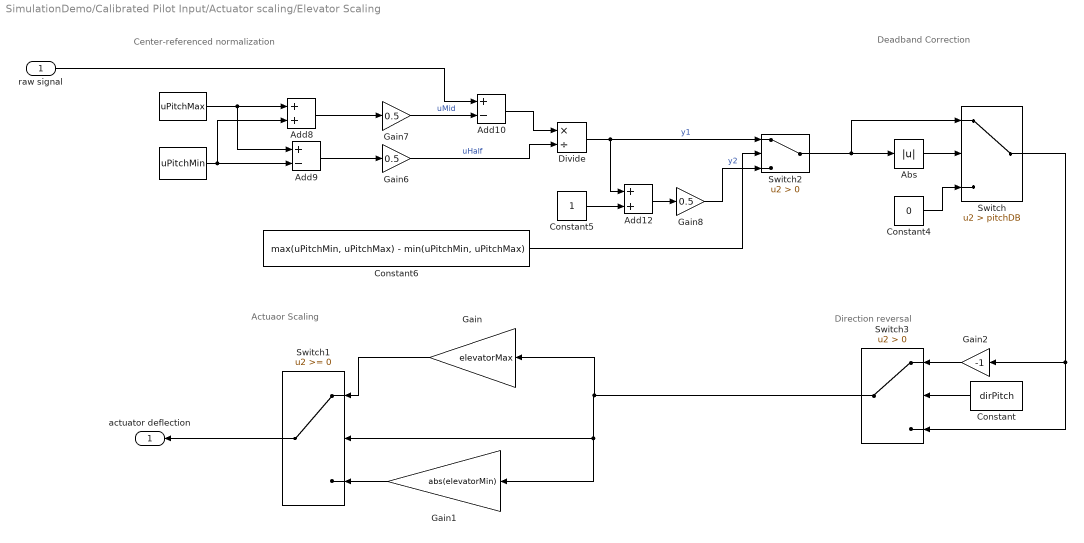
== system SimulationDemo/Calibrated Pilot Input/Actuator scaling/Elevator Scaling ==
  note: Direction reversal
  note: Center-referenced normalization
  note: Deadband Correction
  note: Actuaor Scaling
  raw signal : Inport
  " " : Constant  Value=uPitchMin
  "   " : Constant  Value=uPitchMax
  Abs : Abs  SaturateOnIntegerOverflow=off
  Add10 : Sum  Inputs=+-
  Add12 : Sum
  Add8 : Sum
  Add9 : Sum  Inputs=+-
  Constant : Constant  Value=dirPitch
  Constant4 : Constant  Value=0
  Constant5 : Constant
  Constant6 : Constant  Value=max(uPitchMin, uPitchMax) - min(uPitchMin, uPitchMax)
  Divide : Product  Inputs=*/
  Gain : Gain  Gain=elevatorMax
  Gain1 : Gain  Gain=abs(elevatorMin)
  Gain2 : Gain  Gain=-1
  Gain6 : Gain  Gain=0.5
  Gain7 : Gain  Gain=0.5
  Gain8 : Gain  Gain=0.5
  Switch : Switch  Criteria=u2 > Threshold  Threshold=pitchDB  SaturateOnIntegerOverflow=off  InputSameDT=off
  Switch1 : Switch  SaturateOnIntegerOverflow=off  InputSameDT=off
  Switch2 : Switch  Criteria=u2 > Threshold  SaturateOnIntegerOverflow=off  InputSameDT=off
  Switch3 : Switch  Criteria=u2 > Threshold  SaturateOnIntegerOverflow=off  InputSameDT=off
  actuator deflection : Outport
  wires:
  Add9/1 -> Gain6/1
  "   "/1 -> Add9/1, Add8/1
  Add8/1 -> Gain7/1
  " "/1 -> Add8/2, Add9/2
  raw signal/1 -> Add10/1
  Gain7/1 -> Add10/2  "uMid"
  Add10/1 -> Divide/1
  Gain6/1 -> Divide/2  "uHalf"
  Switch1/1 -> actuator deflection/1
  Divide/1 -> Add12/1, Switch2/1  "y1"
  Constant5/1 -> Add12/2
  Add12/1 -> Gain8/1
  Constant6/1 -> Switch2/2
  Gain8/1 -> Switch2/3  "y2"
  Abs/1 -> Switch/2
  Constant4/1 -> Switch/3
  Switch/1 -> Gain2/1, Switch3/3
  Gain/1 -> Switch1/1
  Gain1/1 -> Switch1/3
  Gain2/1 -> Switch3/1
  Switch3/1 -> Gain1/1, Switch1/2, Gain/1
  Constant/1 -> Switch3/2
  Switch2/1 -> Switch/1, Abs/1

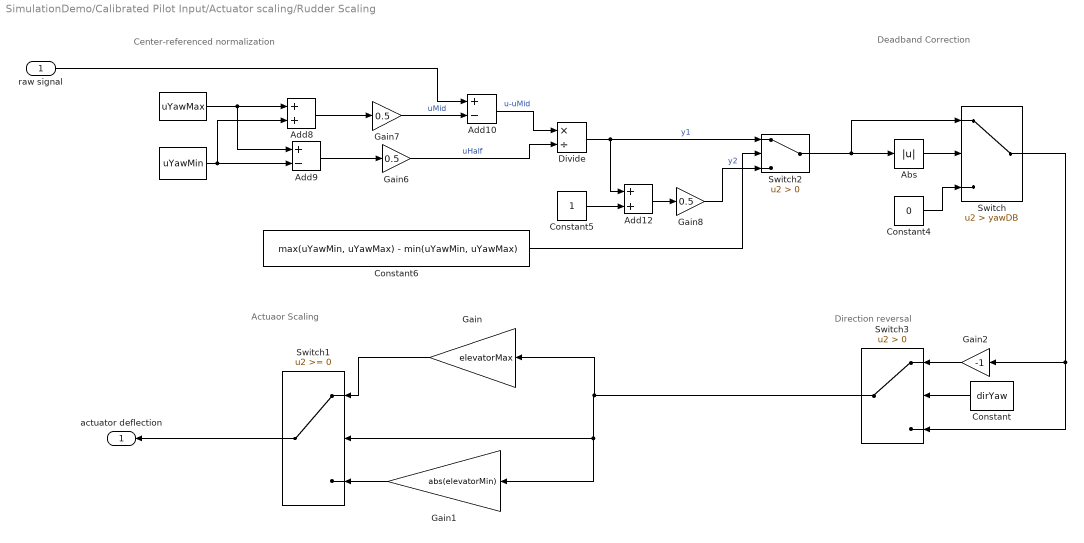
== system SimulationDemo/Calibrated Pilot Input/Actuator scaling/Rudder Scaling ==
  note: Direction reversal
  note: Center-referenced normalization
  note: Deadband Correction
  note: Actuaor Scaling
  raw signal : Inport
  " " : Constant  Value=uYawMin
  "   " : Constant  Value=uYawMax
  Abs : Abs  SaturateOnIntegerOverflow=off
  Add10 : Sum  Inputs=+-
  Add12 : Sum
  Add8 : Sum
  Add9 : Sum  Inputs=+-
  Constant : Constant  Value=dirYaw
  Constant4 : Constant  Value=0
  Constant5 : Constant
  Constant6 : Constant  Value=max(uYawMin, uYawMax) - min(uYawMin, uYawMax)
  Divide : Product  Inputs=*/
  Gain : Gain  Gain=elevatorMax
  Gain1 : Gain  Gain=abs(elevatorMin)
  Gain2 : Gain  Gain=-1
  Gain6 : Gain  Gain=0.5
  Gain7 : Gain  Gain=0.5
  Gain8 : Gain  Gain=0.5
  Switch : Switch  Criteria=u2 > Threshold  Threshold=yawDB  SaturateOnIntegerOverflow=off  InputSameDT=off
  Switch1 : Switch  SaturateOnIntegerOverflow=off  InputSameDT=off
  Switch2 : Switch  Criteria=u2 > Threshold  SaturateOnIntegerOverflow=off  InputSameDT=off
  Switch3 : Switch  Criteria=u2 > Threshold  SaturateOnIntegerOverflow=off  InputSameDT=off
  actuator deflection : Outport
  wires:
  Add9/1 -> Gain6/1
  "   "/1 -> Add9/1, Add8/1
  Add8/1 -> Gain7/1
  " "/1 -> Add8/2, Add9/2
  raw signal/1 -> Add10/1
  Gain7/1 -> Add10/2  "uMid"
  Add10/1 -> Divide/1  "u-uMid"
  Gain6/1 -> Divide/2  "uHalf"
  Switch1/1 -> actuator deflection/1
  Divide/1 -> Add12/1, Switch2/1  "y1"
  Constant5/1 -> Add12/2
  Add12/1 -> Gain8/1
  Constant6/1 -> Switch2/2
  Gain8/1 -> Switch2/3  "y2"
  Abs/1 -> Switch/2
  Constant4/1 -> Switch/3
  Switch/1 -> Gain2/1, Switch3/3
  Gain/1 -> Switch1/1
  Gain1/1 -> Switch1/3
  Gain2/1 -> Switch3/1
  Switch3/1 -> Gain1/1, Switch1/2, Gain/1
  Constant/1 -> Switch3/2
  Switch2/1 -> Switch/1, Abs/1

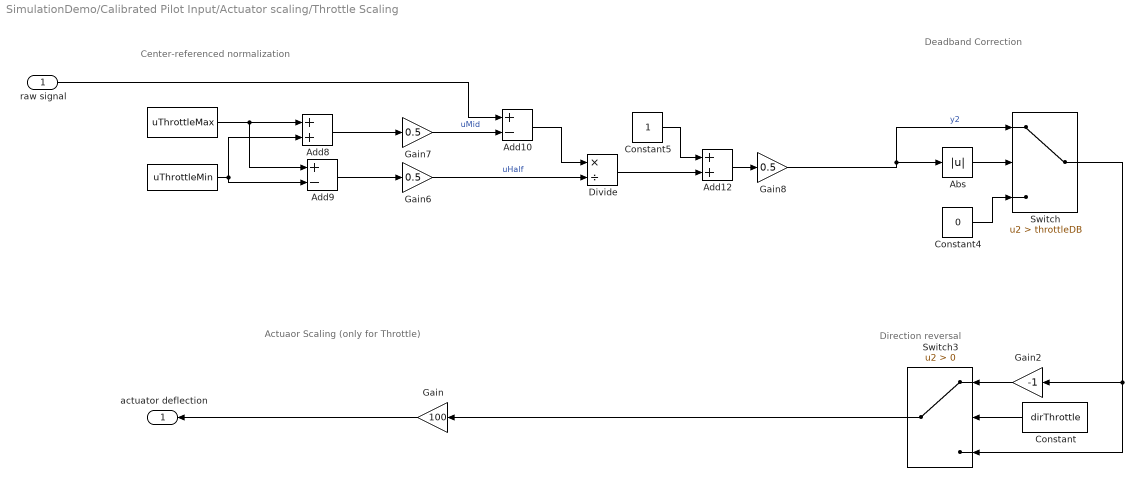
== system SimulationDemo/Calibrated Pilot Input/Actuator scaling/Throttle Scaling ==
  note: Direction reversal
  note: Center-referenced normalization
  note: Deadband Correction
  note: Actuaor Scaling (only for Throttle)
  raw signal : Inport
  " " : Constant  Value=uThrottleMin
  "   " : Constant  Value=uThrottleMax
  Abs : Abs  SaturateOnIntegerOverflow=off
  Add10 : Sum  Inputs=+-
  Add12 : Sum
  Add8 : Sum
  Add9 : Sum  Inputs=+-
  Constant : Constant  Value=dirThrottle
  Constant4 : Constant  Value=0
  Constant5 : Constant
  Divide : Product  Inputs=*/
  Gain : Gain  Gain=100
  Gain2 : Gain  Gain=-1
  Gain6 : Gain  Gain=0.5
  Gain7 : Gain  Gain=0.5
  Gain8 : Gain  Gain=0.5
  Switch : Switch  Criteria=u2 > Threshold  Threshold=throttleDB  SaturateOnIntegerOverflow=off  InputSameDT=off
  Switch3 : Switch  Criteria=u2 > Threshold  SaturateOnIntegerOverflow=off  InputSameDT=off
  actuator deflection : Outport
  wires:
  Add9/1 -> Gain6/1
  "   "/1 -> Add9/1, Add8/1
  Add8/1 -> Gain7/1
  " "/1 -> Add9/2, Add8/2
  raw signal/1 -> Add10/1
  Gain7/1 -> Add10/2  "uMid"
  Add10/1 -> Divide/1
  Gain6/1 -> Divide/2  "uHalf"
  Add12/1 -> Gain8/1
  Gain8/1 -> Switch/1, Abs/1  "y2"
  Abs/1 -> Switch/2
  Constant4/1 -> Switch/3
  Switch/1 -> Gain2/1, Switch3/3
  Gain2/1 -> Switch3/1
  Constant/1 -> Switch3/2
  Gain/1 -> actuator deflection/1
  Switch3/1 -> Gain/1
  Constant5/1 -> Add12/1
  Divide/1 -> Add12/2

== system SimulationDemo/Environment/Environment Source/Custom Environment Parameters ==
  Custom Elevation : Constant  Value=envCustomSource.Location.Elevation_MSL_m
  Custom ISA Deviation : Constant  Value=envCustomSource.Atmosphere.ISA_Deviation_C
  Custom Latitude : Constant  Value=envCustomSource.Location.Latitude_deg
  Custom Longitude : Constant  Value=envCustomSource.Location.Longitude_deg
  Latitude_deg : Outport
  Longitude_deg : Outport  Port=2
  Elevation_MSL_m : Outport  Port=3
  ISA_Deviation_C : Outport  Port=4
  wires:
  Custom Latitude/1 -> Latitude_deg/1
  Custom Longitude/1 -> Longitude_deg/1
  Custom Elevation/1 -> Elevation_MSL_m/1
  Custom ISA Deviation/1 -> ISA_Deviation_C/1

== system SimulationDemo/Environment/Environment Source/Preset Environment Parameters ==
  Preset Elevation : Constant  Value=envPresetSource.Location.Elevation_MSL_m
  Preset ISA Deviation : Constant  Value=envPresetSource.Atmosphere.ISA_Deviation_C
  Preset Latitude : Constant  Value=envPresetSource.Location.Latitude_deg
  Preset Longitude : Constant  Value=envPresetSource.Location.Longitude_deg
  Latitude_deg : Outport
  Longitude_deg : Outport  Port=2
  Elevation_MSL_m : Outport  Port=3
  ISA_Deviation_C : Outport  Port=4
  wires:
  Preset Latitude/1 -> Latitude_deg/1
  Preset Longitude/1 -> Longitude_deg/1
  Preset Elevation/1 -> Elevation_MSL_m/1
  Preset ISA Deviation/1 -> ISA_Deviation_C/1

== system SimulationDemo/Visualizations/Flight parameters /Scope Plot ==
  In1 : Inport
  Bus Selector : BusSelector  OutputSignals=Ve,Vb,Xe,Euler_angles,wb,Actuator deflections
  Bus Selector1 : BusSelector  OutputSignals=Aileron,Elevator,Rudder,Throttle
  Demux{,1,3..4} (4 alike) : Demux  Outputs=3
  Position and Attitude : Scope  NumInputPorts=6
      settings: TimeSpan=10  ActiveDisplayYMinimum=-2.53158999549568  ActiveDisplayYMaximum=6.1729039354737454
  Radians to Degrees1 : simulink_extras/Transformations/Radians to Degrees  Commented=through
  Radians to Degrees2 : simulink_extras/Transformations/Radians to Degrees
  "Velocities, Rates and Controls" : Scope  NumInputPorts=10
      settings: ActiveDisplayYMinimum=10.4194717708245  ActiveDisplayYMaximum=18.842280914352834
  wires:
  Bus Selector1/4 -> "Velocities, Rates and Controls"/10  "<Throttle>"
  Bus Selector1/3 -> "Velocities, Rates and Controls"/9  "<Rudder>"
  Bus Selector1/2 -> "Velocities, Rates and Controls"/8  "<Elevator>"
  Bus Selector1/1 -> "Velocities, Rates and Controls"/7  "<Aileron>"
  Demux1/3 -> "Velocities, Rates and Controls"/6  "r"
  Demux1/2 -> "Velocities, Rates and Controls"/5  "q"
  Demux1/1 -> "Velocities, Rates and Controls"/4  "p"
  Demux/3 -> "Velocities, Rates and Controls"/3  "w"
  Demux/2 -> "Velocities, Rates and Controls"/2  "v"
  Demux/1 -> "Velocities, Rates and Controls"/1  "u"
  Demux3/3 -> Position and Attitude/6  "Alt"
  Demux3/2 -> Position and Attitude/4  "Y"
  Demux3/1 -> Position and Attitude/2  "X"
  Demux4/3 -> Position and Attitude/5  "Psy"
  Demux4/2 -> Position and Attitude/3  "Theta"
  Demux4/1 -> Position and Attitude/1  "Phi"
  Bus Selector/2 -> Demux/1  "<Vb>"
  Bus Selector/6 -> Bus Selector1/1  "<Actuator deflections>"
  In1/1 -> Bus Selector/1
  Radians to Degrees2/1 -> Demux4/1  "Euler Angles"
  Bus Selector/5 -> Radians to Degrees1/1  "<wb>"
  Bus Selector/3 -> Demux3/1  "<Xe>"
  Radians to Degrees1/1 -> Demux1/1  "Euler Angles"
  Bus Selector/4 -> Radians to Degrees2/1  "<Euler_angles>"

== system SimulationDemo/Visualizations/Trajectory Visualization/3D Animation ==
  AC States : Inport
  Bus Selector : BusSelector  OutputSignals=Xe,q
  UAV_Animation : uavutilslib/UAV Animation  NumUAV=1  DynamicUAVConfig=off  UAVType=FixedWing  UAVSize=1  UAVColor=[1 0 0]  UAVTrajectoryAlpha=1  InertialZDirection=Down  RotationFormat=Quaternion  DrawMarkers=off  SampleTime=-1
  wires:
  Bus Selector/1 -> UAV_Animation/1  "<Xe>"
  Bus Selector/2 -> UAV_Animation/2  "<q>"
  AC States/1 -> Bus Selector/1
